simulink model "fangzhen"  (R2018b)
settings: Solver=ode45  StartTime=0.0  StopTime=10  FixedStep=0.0002  MaxStep=1/5000/25  MinStep=1/5000/100  RelTol=2e-4  EnableMultiTasking=on
libraries: powerlib_meascontrol x6, powerlib x5, simulink x4, powerlib_extras x1
(part 1 of 2)
settings Model: Creator=Administrator  LastModifiedBy=ThinkPad
settings DataIOCC: LimitDataPoints=on  SaveFormat=Array  SignalLoggingSaveFormat=ModelDataLogs
settings OptimizationCC: ExpressionDepthLimit=2147483647  LifeSpan=inf
settings DebuggingCC: UnderspecifiedInitializationDetection=Classic  MergeDetectMultiDrivingBlocksExec=none  SolverPrmCheckMsg=warning  FcnCallInpInsideContextMsg=warning  UnconnectedInputMsg=none  UnconnectedOutputMsg=none  UnconnectedLineMsg=none  StateNameClashWarn=warning  LibraryContextMissingDiagnostic=none  SFUnexpectedBacktrackingDiag=warning  SFNoUnconditionalDefaultTransitionDiag=warning  SFExecutionAtInitializationDiag=none
settings HardwareCC: ProdBitPerPointer=32  ProdBitPerSizeT=32  ProdBitPerPtrDiffT=32  ProdLargestAtomicFloat=None  ProdIntDivRoundTo=Undefined  ProdEndianess=Unspecified  ProdWordSize=32  ProdHWDeviceType=32-bit Generic
settings ModelReferenceCC: PropagateSignalLabelsOutOfModel=off
settings SFSimCC: SimUseLocalCustomCode=off
settings RTWCC: RTWUseLocalCustomCode=off
settings CodeAppCC: StateflowObjectComments=on
settings GRTTargetCC: TargetLangStandard=C89/C90 (ANSI)  GeneratePreprocessorConditionals=Disable all
settings ConfigComp: CovMetricSettings=dw  CovHtmlReporting=on  CovSaveCumulativeToWorkspaceVar=on  CovSaveSingleToWorkspaceVar=on  CovExternalEMLEnable=off
settings SimscapeCC: SimscapeNormalizeSystem=off

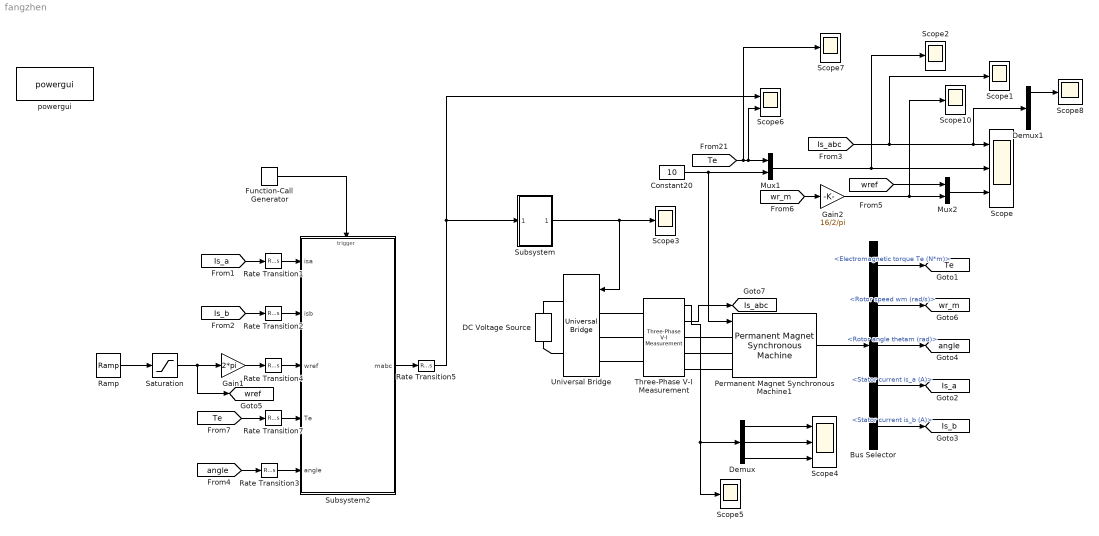
== system fangzhen ==
  Bus Selector : BusSelector  OutputSignals=Electromagnetic torque Te (N*m),Rotor speed wm (rad/s),Rotor angle thetam (rad),Stator current is_a (A),Stator current is_b (A)
  Constant20 : Constant  Value=10  OutDataTypeStr=double
  DC Voltage Source : powerlib/Electrical Sources/DC Voltage Source  Amplitude=400  Measurements=None
      settings: SourceProductName=Simscape Electrical
  Demux : Demux  Outputs=3
  Demux1 : Demux  Outputs=3
  Function-Call Generator : simulink/Ports & Subsystems/Function-Call Generator  sample_time=1/5000  numberOfIterations=1
  Gain1 : Gain  Gain=2*pi
  Gain2 : Gain  Gain=16/2/pi
  Mux1 : Mux  Inputs=2
  Mux2 : Mux  Inputs=2
  Permanent Magnet Synchronous Machine1 : powerlib/Machines/Permanent Magnet Synchronous Machine  NbPhases=3  FluxDistribution=Sinusoidal  RotorType=Round  MechanicalLoad=Torque Tm  PresetModel=No  ShowDetailedParameters=on  MeasurementBus=off  Resistance=0.4  Inductance=8.5e-3  dqInductances=[8.5e-3,8.5e-3]  La=0.004  MachineConstant=Torque Constant (N.m / A_peak)  Flux=0.56178  VoltageCst=1630.3396  TorqueCst=13.4828  Flat=120  Mechanical=[0.00062 0.0003035 16 0]  PolePairs=16  InitialConditions=[0,0, 0,0]  InitialConditions5ph=[0 0 0 0 0 0]  TsPowergui=0  TsBlock=-1  RefAngle=Aligned with phase A axis (original Park)
  Ramp : simulink/Sources/Ramp  slope=30/0.1  start=0  InitialOutput=0
  Rate Transition{1..5,7} (6 alike) : RateTransition  Integrity=off
  Saturation : Saturate  UpperLimit=10  LowerLimit=0
  Scope : Scope  NumInputPorts=3
  Scope{1..3,5,7..8,10} (7 alike) : Scope
  Scope4 : Scope  NumInputPorts=3
  Scope6 : Scope  NumInputPorts=2
  Subsystem : Subsystem
  Subsystem2 : Subsystem
  Three-Phase V-I Measurement : powerlib/Measurements/Three-Phase V-I Measurement  VoltageMeasurement=phase-to-phase  SetLabelV=off  LabelV=Vabc  Vpu=off  VpuLL=off  CurrentMeasurement=yes  SetLabelI=off  LabelI=Iabc  Ipu=off  Pbase=100e6  Vbase=500e3  OutputType=Complex  PhasorSimulation=off  PSBequivalent=0
      settings: SourceProductName=Simscape Electrical
  Universal Bridge : powerlib/Power Electronics/Universal Bridge  Arms=3  SnubberResistance=1e5  SnubberCapacitance=inf  Device=IGBT / Diodes  Ron=1e-3  Lon=0  ForwardVoltages="[  3  2  ]"  ForwardVoltage=0  GTOparameters=[ 10e-6 , 20e-6 ]  IGBTparameters=[ 1e-6 , 2e-6 ]  Measurements=All voltages and currents  Measurements_2=None  converterType=Rectifier
      settings: SourceProductName=Simscape Electrical
  powergui : powerlib/powergui  Priority=2  SimulationMode=Discrete  SampleTime=1/5000/30/20  frequency=60  Iterations=50  frequencyindice=0  Pbase=100e6  ErrMax=1e-4  UnitsV=kV  UnitsW=MW  buscounter=0  FunctionMessages=off  echomessages=off  EnableUseOfTLC=off  CurrentSourceSwitches=off  DisableSnubberDevices=off  DisableRonSwitches=off  DisableVfSwitches=off  DisplayEquations=off  SolverType=Tustin  Interpol=off  ExternalGateDelay=off  methode=off  Ts=0  x0status=blocks  SPID=off  SwTol=0  HookPort=off  RestoreLinks=warning  ResistiveCurrentMeasurement=off  Frange=[0:2:500]  Ylog=off  Xlog=on  ShowGrid=off  save=off  variable=ZData  structure=TEwu  ZoomFFT=off  StartTime=9  cycles=8  DisplayStyle=1  fundamental=10  FreqAxis=on  MaxFrequency=100  frequencyindicesteady=1  RmsSteady=1  display=off
  tag scope: Is_a=global, Is_abc=global, Is_b=global, Te=global, angle=global, wr_m=global, wref=global
  wires:
  [wref] -> Mux2/1
  Rate Transition7/1 -> Subsystem2/4(Te)
  Gain2/1 -> Mux2/2, Scope10/1
  Three-Phase V-I Measurement/2 -> [Is_abc]
  [angle] -> Rate Transition3/1
  Rate Transition2/1 -> Subsystem2/2(isb)
  Bus Selector/2 -> [wr_m]  "<Rotor speed wm (rad/s)>"
  Demux/1 -> Scope4/1
  Ramp/1 -> Saturation/1
  Demux/2 -> Scope4/2
  Gain1/1 -> Rate Transition4/1
  Bus Selector/5 -> [Is_b]  "<Stator current is_b (A)>"
  [Is_b] -> Rate Transition2/1
  Mux2/1 -> Scope/3
  Rate Transition5/1 -> Subsystem/1(In1), Scope6/1
  Rate Transition1/1 -> Subsystem2/1(isa)
  Rate Transition4/1 -> Subsystem2/3(wref)
  Bus Selector/1 -> [Te]  "<Electromagnetic torque Te (N*m)>"
  [wr_m] -> Gain2/1
  [Te] -> Scope7/1, Mux1/1, Scope6/2
  Three-Phase V-I Measurement/1 -> Demux/1, Scope5/1
  [Te] -> Rate Transition7/1
  Bus Selector/3 -> [angle]  "<Rotor angle thetam (rad)>"
  [Is_a] -> Rate Transition1/1
  Permanent Magnet Synchronous Machine1/1 -> Bus Selector/1
  Constant20/1 -> Permanent Magnet Synchronous Machine1/1, Mux1/2
  Saturation/1 -> Gain1/1, [wref]
  Mux1/1 -> Scope2/1, Scope/2
  Rate Transition3/1 -> Subsystem2/5(angle)
  Bus Selector/4 -> [Is_a]  "<Stator current is_a (A)>"
  [Is_abc] -> Scope1/1, Demux1/1, Scope/1
  Demux/3 -> Scope4/3
  Subsystem/1(Out1) -> Universal Bridge/1, Scope3/1
  Function-Call Generator/1 -> Subsystem2/Trigger
  Subsystem2/1(mabc) -> Rate Transition5/1
  Demux1/1 -> Scope8/1
  connections:
  Universal Bridge/LConn2 -- Three-Phase V-I Measurement/LConn2
  Universal Bridge/LConn3 -- Three-Phase V-I Measurement/LConn3
  Universal Bridge/LConn1 -- Three-Phase V-I Measurement/LConn1
  DC Voltage Source/RConn1 -- Universal Bridge/RConn1
  Universal Bridge/RConn2 -- DC Voltage Source/LConn1
  Permanent Magnet Synchronous Machine1/LConn2 -- Three-Phase V-I Measurement/RConn2
  Three-Phase V-I Measurement/RConn3 -- Permanent Magnet Synchronous Machine1/LConn3
  Permanent Magnet Synchronous Machine1/LConn1 -- Three-Phase V-I Measurement/RConn1

== system fangzhen/Subsystem ==
  In1 : Inport
  Demux1 : Demux  Outputs=6
  Mux : Mux  Inputs=6
  On Delay{,1..5} (6 alike) : powerlib_meascontrol/Logic/On Delay  DelayType=On delay  delay=5e-6  ic=0  Ts=0
      settings: SourceProductName=Simscape Power Systems
  PWM Generator : powerlib_extras/Control  Blocks/PWM Generator  GeneratorMode="3-arm  bridge (6 pulses)"  Fc=5000  Internal=off  mIndex=0.4  Freq=60  Phase=0
  Scope{1..3,7..9} (6 alike) : Scope  NumInputPorts=2
  Out1 : Outport
  wires:
  Demux1/6 -> On Delay5/1, Scope7/2
  Demux1/3 -> On Delay2/1, Scope8/1
  In1/1 -> PWM Generator/1
  Demux1/4 -> On Delay3/1, Scope8/2
  PWM Generator/1 -> Demux1/1
  Demux1/2 -> On Delay1/1, Scope9/2
  Demux1/5 -> On Delay4/1, Scope7/1
  Demux1/1 -> Scope9/1, On Delay/1
  On Delay/1 -> Scope3/1, Mux/1
  On Delay1/1 -> Mux/2, Scope3/2
  On Delay2/1 -> Scope2/1, Mux/3
  On Delay3/1 -> Scope2/2, Mux/4
  On Delay4/1 -> Scope1/1, Mux/5
  On Delay5/1 -> Scope1/2, Mux/6
  Mux/1 -> Out1/1

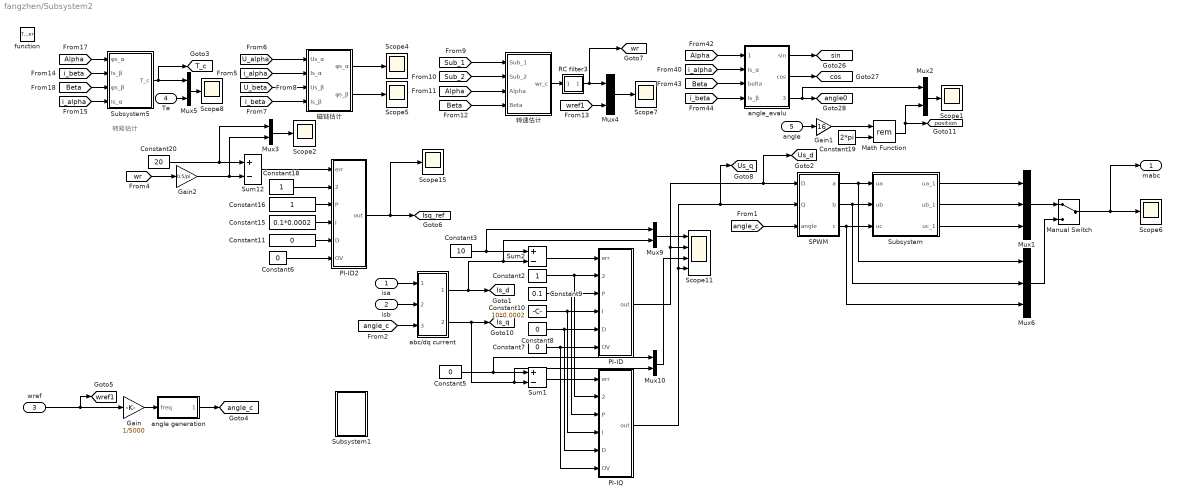
== system fangzhen/Subsystem2 ==
  note: 转矩估计
  isa : Inport
  isb : Inport  Port=2
  wref : Inport  Port=3
  Te : Inport  Port=4
  angle : Inport  Port=5
  function : TriggerPort  TriggerType=function-call  VariantControl=(inherit)
  Constant10 : Constant  Value=10*0.0002  OutDataTypeStr=double
  Constant{5..8,11} (5 alike) : Constant  Value=0  OutDataTypeStr=double
  Constant15 : Constant  Value=0.1*0.0002  OutDataTypeStr=double
  Constant16 : Constant  OutDataTypeStr=double
  Constant18 : Constant  OutDataTypeStr=double
  Constant19 : Constant  Value=2*pi  OutDataTypeStr=double
  Constant2 : Constant  OutDataTypeStr=double
  Constant20 : Constant  Value=20  OutDataTypeStr=double
  Constant3 : Constant  Value=10  OutDataTypeStr=double
  Constant9 : Constant  Value=0.1  OutDataTypeStr=double
  Gain : Gain  Gain=1/5000
  Gain1 : Gain  Gain=16
  Gain2 : Gain  Gain=0.5/pi
  Manual Switch : ManualSwitch
  Math Function : Math  Operator=rem  SaturateOnIntegerOverflow=on
  Mux1 : Mux  Inputs=3
  Mux{2..5,9..10} (6 alike) : Mux  Inputs=2
  Mux6 : Mux  Inputs=3
  PI-ID : Subsystem  mask{ermax=1000, ermin=-1000, max=1, min=-1}
      mask prompts: ermax "Err max limit"; ermin "Err min limit"; max "Output max limit"; min "Output min limit"
  PI-ID2 : Subsystem  mask{ermax=10, ermin=-10, max=5, min=0}
      mask prompts: ermax "Err max limit"; ermin "Err min limit"; max "Output max limit"; min "Output min limit"
  PI-IQ : Subsystem  mask{ermax=100, ermin=-100, max=1, min=-1}
      mask prompts: ermax "Err max limit"; ermin "Err min limit"; max "Output max limit"; min "Output min limit"
  RC filter3 : Subsystem  mask{a=1/4}
      mask prompts: a "Time Constant"
  SPWM : Subsystem
  Scope{1..2,4..8,15} (8 alike) : Scope
  Scope11 : Scope  NumInputPorts=4
  Subsystem : Subsystem
  Subsystem1 : Subsystem
  Subsystem5 : Subsystem
  Sum1 : Sum  Inputs=+-
  Sum12 : Sum  Inputs=+-
  Sum2 : Sum  Inputs=+-
  abc/dq current : Subsystem
  angle generation : Subsystem
  angle_evalu : Subsystem
  磁链估计 : Subsystem
  转速估计 : Subsystem
  mabc : Outport
  tag scope: Is_d=global, Is_q=global, Isq_ref=global, T_c=global, Us_d=global, Us_q=global, angle0=global, angle_c=global, cos=global, position=global, sin=global, wr=global, wref1=global
  wires:
  Mux1/1 -> Manual Switch/1
  isa/1 -> abc/dq current/1(iga)
  abc/dq current/1(igd) -> Sum2/2, Mux9/2, [Is_d]
  abc/dq current/2(igq) -> Sum1/2, Mux10/2, [Is_q]
  Constant7/1 -> PI-ID/6(OV), PI-IQ/6(OV)
  Constant8/1 -> PI-ID/5(D), PI-IQ/5(D)
  Constant10/1 -> PI-ID/4(I), PI-IQ/4(I)
  Constant9/1 -> PI-ID/3(P), PI-IQ/3(P)
  Sum2/1 -> PI-ID/1(err)
  Constant2/1 -> PI-ID/2(reset), PI-IQ/2(reset)
  PI-ID/1(out) -> Scope11/2, [Us_d], SPWM/1(D)
  PI-IQ/1(out) -> Scope11/4, [Us_q], SPWM/2(Q)
  Sum1/1 -> PI-IQ/1(err)
  [angle_c] -> SPWM/3(angle)
  Gain/1 -> angle generation/1(freq)
  Mux9/1 -> Scope11/1
  Mux10/1 -> Scope11/3
  isb/1 -> abc/dq current/2(igb)
  angle generation/1(angle_0) -> [angle_c]
  [angle_c] -> abc/dq current/3(angle)
  wref/1 -> Gain/1, [wref1]
  [Beta] -> 转速估计/4(Beta)
  [Alpha] -> 转速估计/3(Alpha)
  [Sub_2] -> 转速估计/2(Sub_2)
  [Sub_1] -> 转速估计/1(Sub_1)
  转速估计/1(wr_c) -> RC filter3/1(x)
  Mux4/1 -> Scope7/1
  [U_alpha] -> 磁链估计/1(Us_α)
  [i_alpha] -> 磁链估计/2(Is_α)
  [U_beta] -> 磁链估计/3(Us_β)
  [i_beta] -> 磁链估计/4(Is_β)
  磁链估计/2(φs_β) -> Scope5/1
  磁链估计/1(φs_α) -> Scope4/1
  [Alpha] -> Subsystem5/1(φs_α)
  [Beta] -> Subsystem5/3(φs_β)
  [i_beta] -> Subsystem5/2(Is_β)
  [i_alpha] -> Subsystem5/4(Is_α)
  Subsystem5/1(T_c) -> Mux5/1, [T_c]
  Mux5/1 -> Scope8/1
  Te/1 -> Mux5/2
  RC filter3/1(y) -> [wr], Mux4/1
  [wref1] -> Mux4/2
  [wr] -> Gain2/1
  Constant20/1 -> Sum12/1, Mux3/1
  Sum12/1 -> PI-ID2/1(err)
  Constant18/1 -> PI-ID2/2(reset)
  Constant16/1 -> PI-ID2/3(P)
  Constant15/1 -> PI-ID2/4(I)
  Constant11/1 -> PI-ID2/5(D)
  Constant6/1 -> PI-ID2/6(OV)
  PI-ID2/1(out) -> Scope15/1, [Isq_ref]
  Constant5/1 -> Sum1/1, Mux10/1
  Constant3/1 -> Sum2/1, Mux9/1
  [Alpha] -> angle_evalu/1(alpha)
  [Beta] -> angle_evalu/3(belta)
  [i_beta] -> angle_evalu/4(Is_β)
  [i_alpha] -> angle_evalu/2(Is_α)
  angle_evalu/1(sin) -> [sin]
  angle_evalu/2(cos) -> [cos]
  angle_evalu/3(angle_0) -> [angle0], Mux2/1
  Mux2/1 -> Scope1/1
  angle/1 -> Gain1/1
  Mux3/1 -> Scope2/1
  Constant19/1 -> Math Function/2
  Gain1/1 -> Math Function/1
  Math Function/1 -> Mux2/2, [position]
  Gain2/1 -> Sum12/2, Mux3/2
  SPWM/1(a) -> Subsystem/1(ua), Mux6/1
  SPWM/2(b) -> Subsystem/2(ub), Mux6/2
  SPWM/3(c) -> Subsystem/3(uc), Mux6/3
  Subsystem/1(ua_1) -> Mux1/1
  Subsystem/3(uc_1) -> Mux1/3
  Subsystem/2(ub_1) -> Mux1/2
  Mux6/1 -> Manual Switch/2
  Manual Switch/1 -> Scope6/1, mabc/1

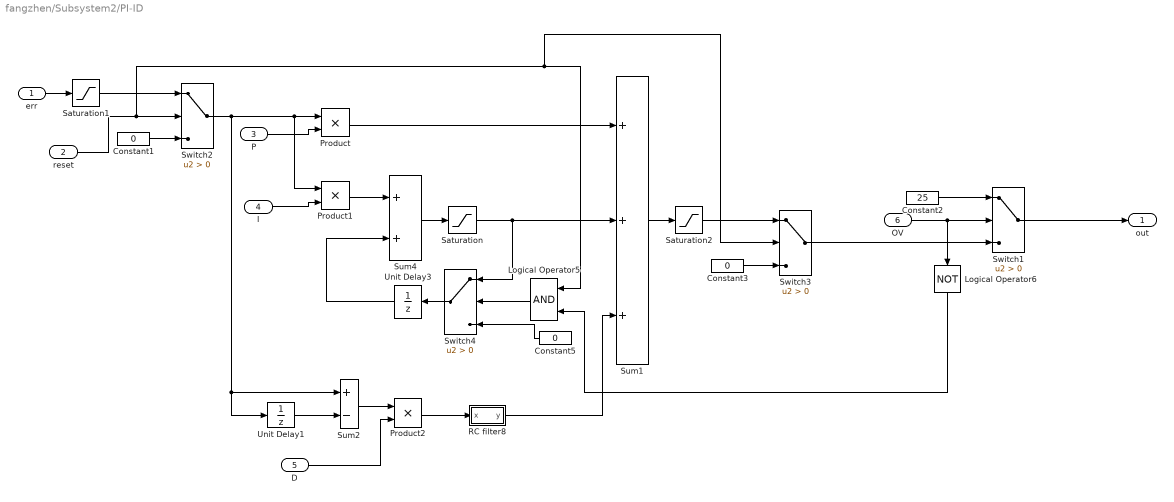
== system fangzhen/Subsystem2/PI-ID ==
  err : Inport
  reset : Inport  Port=2
  P : Inport  Port=3
  I : Inport  Port=4
  D : Inport  Port=5
  OV : Inport  Port=6
  Constant1 : Constant  Value=0  OutDataTypeStr=Inherit: Inherit via back propagation
  Constant2 : Constant  Value=25  OutDataTypeStr=Inherit: Inherit via back propagation
  Constant3 : Constant  Value=0  OutDataTypeStr=Inherit: Inherit via back propagation
  Constant5 : Constant  Value=0  OutDataTypeStr=Inherit: Inherit via back propagation
  Logical Operator5 : Logic  AllPortsSameDT=off  OutDataTypeStr=boolean
  Logical Operator6 : Logic  Operator=NOT  AllPortsSameDT=off  OutDataTypeStr=boolean
  Product : Product  RndMeth=Zero
  Product1 : Product  RndMeth=Zero
  Product2 : Product  RndMeth=Zero
  RC filter8 : Subsystem  mask{a=0.4}
      mask prompts: a "Time Constant"
  Saturation : Saturate  UpperLimit=max  LowerLimit=min  LinearizeAsGain=off  ZeroCross=off  OutDataTypeStr=double
  Saturation1 : Saturate  UpperLimit=ermax  LowerLimit=ermin  LinearizeAsGain=off  ZeroCross=off  OutDataTypeStr=double
  Saturation2 : Saturate  UpperLimit=max  LowerLimit=min  LinearizeAsGain=off  ZeroCross=off  OutDataTypeStr=double
  Sum1 : Sum  Inputs=+++
  Sum2 : Sum  Inputs=+-
  Sum4 : Sum
  Switch{1..4} (4 alike) : Switch  Criteria=u2 > Threshold  SaturateOnIntegerOverflow=on  InputSameDT=on
  Unit Delay1 : UnitDelay  SampleTime=-1
  Unit Delay3 : UnitDelay  SampleTime=-1
  out : Outport
  wires:
  Logical Operator6/1 -> Logical Operator5/2
  Logical Operator5/1 -> Switch4/2
  RC filter8/1(y) -> Sum1/3
  Constant3/1 -> Switch3/3
  Switch3/1 -> Switch1/3
  Saturation2/1 -> Switch3/1
  Switch1/1 -> out/1
  OV/1 -> Logical Operator6/1, Switch1/2
  Constant2/1 -> Switch1/1
  Sum1/1 -> Saturation2/1
  Product2/1 -> RC filter8/1(x)
  Unit Delay1/1 -> Sum2/2
  D/1 -> Product2/2
  Sum2/1 -> Product2/1
  Switch4/1 -> Unit Delay3/1
  Unit Delay3/1 -> Sum4/2
  Saturation/1 -> Switch4/1, Sum1/2
  Sum4/1 -> Saturation/1
  Product1/1 -> Sum4/1
  I/1 -> Product1/2
  Product/1 -> Sum1/1
  Saturation1/1 -> Switch2/1
  err/1 -> Saturation1/1
  Constant1/1 -> Switch2/3
  reset/1 -> Logical Operator5/1, Switch3/2, Switch2/2
  Switch2/1 -> Unit Delay1/1, Sum2/1, Product1/1, Product/1
  P/1 -> Product/2
  Constant5/1 -> Switch4/3

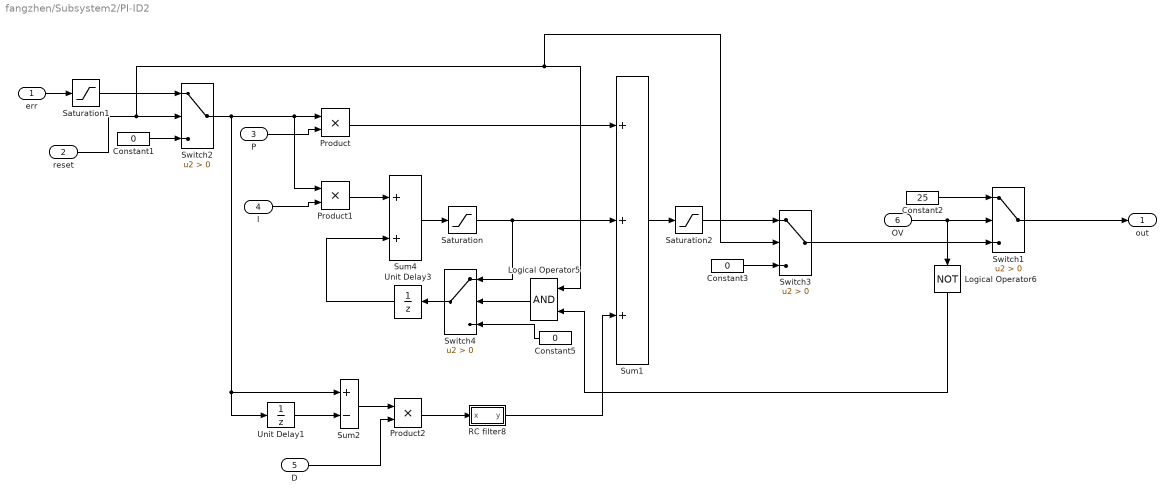
== system fangzhen/Subsystem2/PI-ID2 ==
  err : Inport
  reset : Inport  Port=2
  P : Inport  Port=3
  I : Inport  Port=4
  D : Inport  Port=5
  OV : Inport  Port=6
  Constant1 : Constant  Value=0  OutDataTypeStr=Inherit: Inherit via back propagation
  Constant2 : Constant  Value=25  OutDataTypeStr=Inherit: Inherit via back propagation
  Constant3 : Constant  Value=0  OutDataTypeStr=Inherit: Inherit via back propagation
  Constant5 : Constant  Value=0  OutDataTypeStr=Inherit: Inherit via back propagation
  Logical Operator5 : Logic  AllPortsSameDT=off  OutDataTypeStr=boolean
  Logical Operator6 : Logic  Operator=NOT  AllPortsSameDT=off  OutDataTypeStr=boolean
  Product : Product  RndMeth=Zero
  Product1 : Product  RndMeth=Zero
  Product2 : Product  RndMeth=Zero
  RC filter8 : Subsystem  mask{a=0.4}
      mask prompts: a "Time Constant"
  Saturation : Saturate  UpperLimit=max  LowerLimit=min  LinearizeAsGain=off  ZeroCross=off  OutDataTypeStr=double
  Saturation1 : Saturate  UpperLimit=ermax  LowerLimit=ermin  LinearizeAsGain=off  ZeroCross=off  OutDataTypeStr=double
  Saturation2 : Saturate  UpperLimit=max  LowerLimit=min  LinearizeAsGain=off  ZeroCross=off  OutDataTypeStr=double
  Sum1 : Sum  Inputs=+++
  Sum2 : Sum  Inputs=+-
  Sum4 : Sum
  Switch{1..4} (4 alike) : Switch  Criteria=u2 > Threshold  SaturateOnIntegerOverflow=on  InputSameDT=on
  Unit Delay1 : UnitDelay  SampleTime=-1
  Unit Delay3 : UnitDelay  SampleTime=-1
  out : Outport
  wires:
  Constant5/1 -> Switch4/3
  P/1 -> Product/2
  Switch2/1 -> Product/1, Product1/1, Sum2/1, Unit Delay1/1
  reset/1 -> Switch2/2, Switch3/2, Logical Operator5/1
  Constant1/1 -> Switch2/3
  err/1 -> Saturation1/1
  Saturation1/1 -> Switch2/1
  Product/1 -> Sum1/1
  I/1 -> Product1/2
  Product1/1 -> Sum4/1
  Sum4/1 -> Saturation/1
  Saturation/1 -> Sum1/2, Switch4/1
  Unit Delay3/1 -> Sum4/2
  Switch4/1 -> Unit Delay3/1
  Sum2/1 -> Product2/1
  D/1 -> Product2/2
  Unit Delay1/1 -> Sum2/2
  Product2/1 -> RC filter8/1(x)
  Sum1/1 -> Saturation2/1
  Constant2/1 -> Switch1/1
  OV/1 -> Switch1/2, Logical Operator6/1
  Switch1/1 -> out/1
  Saturation2/1 -> Switch3/1
  Switch3/1 -> Switch1/3
  Constant3/1 -> Switch3/3
  RC filter8/1(y) -> Sum1/3
  Logical Operator5/1 -> Switch4/2
  Logical Operator6/1 -> Logical Operator5/2

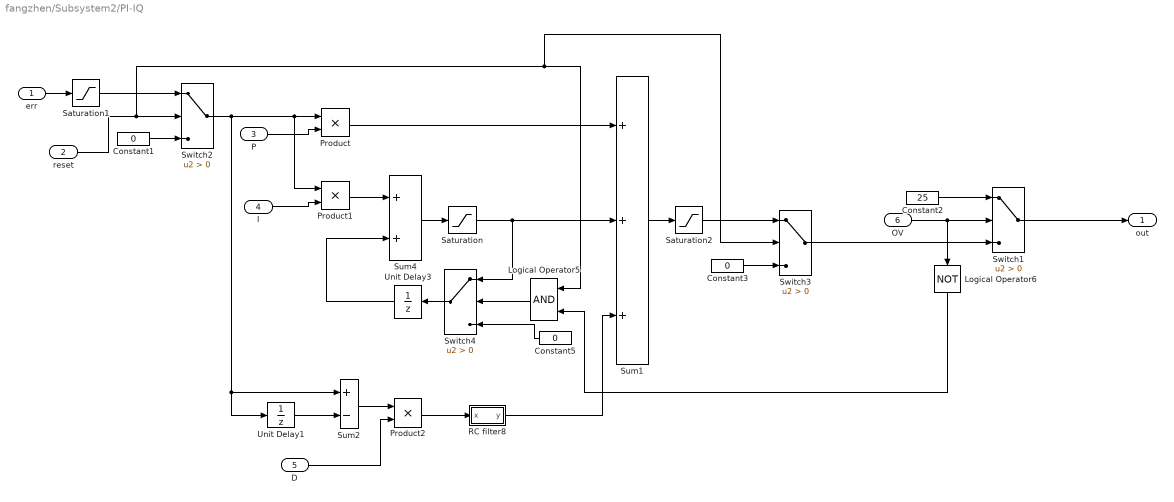
== system fangzhen/Subsystem2/PI-IQ ==
  err : Inport
  reset : Inport  Port=2
  P : Inport  Port=3
  I : Inport  Port=4
  D : Inport  Port=5
  OV : Inport  Port=6
  Constant1 : Constant  Value=0  OutDataTypeStr=Inherit: Inherit via back propagation
  Constant2 : Constant  Value=25  OutDataTypeStr=Inherit: Inherit via back propagation
  Constant3 : Constant  Value=0  OutDataTypeStr=Inherit: Inherit via back propagation
  Constant5 : Constant  Value=0  OutDataTypeStr=Inherit: Inherit via back propagation
  Logical Operator5 : Logic  AllPortsSameDT=off  OutDataTypeStr=boolean
  Logical Operator6 : Logic  Operator=NOT  AllPortsSameDT=off  OutDataTypeStr=boolean
  Product : Product  RndMeth=Zero
  Product1 : Product  RndMeth=Zero
  Product2 : Product  RndMeth=Zero
  RC filter8 : Subsystem  mask{a=0.4}
      mask prompts: a "Time Constant"
  Saturation : Saturate  UpperLimit=max  LowerLimit=min  LinearizeAsGain=off  ZeroCross=off  OutDataTypeStr=double
  Saturation1 : Saturate  UpperLimit=ermax  LowerLimit=ermin  LinearizeAsGain=off  ZeroCross=off  OutDataTypeStr=double
  Saturation2 : Saturate  UpperLimit=max  LowerLimit=min  LinearizeAsGain=off  ZeroCross=off  OutDataTypeStr=double
  Sum1 : Sum  Inputs=+++
  Sum2 : Sum  Inputs=+-
  Sum4 : Sum
  Switch{1..4} (4 alike) : Switch  Criteria=u2 > Threshold  SaturateOnIntegerOverflow=on  InputSameDT=on
  Unit Delay1 : UnitDelay  SampleTime=-1
  Unit Delay3 : UnitDelay  SampleTime=-1
  out : Outport
  wires:
  Constant5/1 -> Switch4/3
  P/1 -> Product/2
  Switch2/1 -> Product/1, Product1/1, Sum2/1, Unit Delay1/1
  reset/1 -> Switch2/2, Switch3/2, Logical Operator5/1
  Constant1/1 -> Switch2/3
  err/1 -> Saturation1/1
  Saturation1/1 -> Switch2/1
  Product/1 -> Sum1/1
  I/1 -> Product1/2
  Product1/1 -> Sum4/1
  Sum4/1 -> Saturation/1
  Saturation/1 -> Sum1/2, Switch4/1
  Unit Delay3/1 -> Sum4/2
  Switch4/1 -> Unit Delay3/1
  Sum2/1 -> Product2/1
  D/1 -> Product2/2
  Unit Delay1/1 -> Sum2/2
  Product2/1 -> RC filter8/1(x)
  Sum1/1 -> Saturation2/1
  Constant2/1 -> Switch1/1
  OV/1 -> Switch1/2, Logical Operator6/1
  Switch1/1 -> out/1
  Saturation2/1 -> Switch3/1
  Switch3/1 -> Switch1/3
  Constant3/1 -> Switch3/3
  RC filter8/1(y) -> Sum1/3
  Logical Operator5/1 -> Switch4/2
  Logical Operator6/1 -> Logical Operator5/2

== system fangzhen/Subsystem2/RC filter3 ==
  x : Inport
  Constant2 : Constant  Value=a  OutDataTypeStr=double
  Constant3 : Constant  Value=1-a  OutDataTypeStr=double
  Divide : Product
  Divide1 : Product
  Sum2 : Sum
  Unit Delay2 : UnitDelay  SampleTime=-1
  y : Outport
  wires:
  Unit Delay2/1 -> Divide1/2
  Sum2/1 -> Unit Delay2/1, y/1
  Divide1/1 -> Sum2/2
  Divide/1 -> Sum2/1
  Constant3/1 -> Divide1/1
  Constant2/1 -> Divide/2
  x/1 -> Divide/1

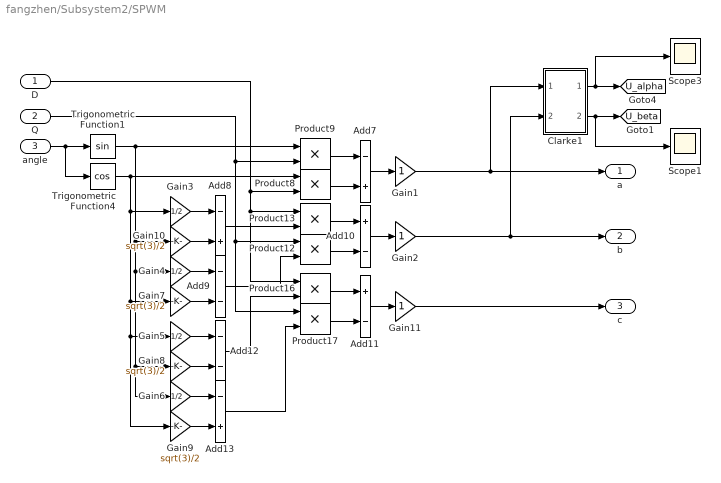
== system fangzhen/Subsystem2/SPWM ==
  D : Inport
  Q : Inport  Port=2
  angle : Inport  Port=3
  Add10 : Sum  Inputs=+-
  Add11 : Sum  Inputs=+-
  Add12 : Sum  Inputs=--
  Add13 : Sum  Inputs=-+
  Add7 : Sum  Inputs=-+
  Add8 : Sum  Inputs=-+
  Add9 : Sum  Inputs=--
  Clarke1 : Subsystem
  Gain1 : Gain
  Gain{7..10} (4 alike) : Gain  Gain=sqrt(3)/2
  Gain11 : Gain
  Gain2 : Gain
  Gain{3..6} (4 alike) : Gain  Gain=1/2
  Product{8..9,12..13,16..17} (6 alike) : Product  RndMeth=Zero
  Scope1 : Scope
  Scope3 : Scope
  Trigonometric Function1 : Trigonometry
  Trigonometric Function4 : Trigonometry  Operator=cos
  a : Outport
  b : Outport  Port=2
  c : Outport  Port=3
  tag scope: U_alpha=global, U_beta=global
  wires:
  angle/1 -> Trigonometric Function1/1, Trigonometric Function4/1
  Trigonometric Function4/1 -> Product8/1, Gain3/1, Gain5/1, Gain9/1, Gain7/1
  Product8/1 -> Add7/2
  Trigonometric Function1/1 -> Product9/1, Gain4/1, Gain6/1, Gain8/1, Gain10/1
  Product9/1 -> Add7/1
  Gain3/1 -> Add8/1
  Gain4/1 -> Add9/1
  Gain7/1 -> Add9/2
  Product13/1 -> Add10/1
  Product12/1 -> Add10/2
  Add8/1 -> Product13/2
  Add9/1 -> Product12/2
  Product16/1 -> Add11/1
  Product17/1 -> Add11/2
  Add12/1 -> Product16/2
  Add13/1 -> Product17/2
  Add7/1 -> Gain1/1
  Add10/1 -> Gain2/1
  Add11/1 -> Gain11/1
  Gain6/1 -> Add13/1
  Gain8/1 -> Add12/2
  Gain5/1 -> Add12/1
  Gain9/1 -> Add13/2
  Gain10/1 -> Add8/2
  D/1 -> Product8/2, Product13/1, Product16/1
  Q/1 -> Product9/2, Product12/1, Product17/1
  Gain1/1 -> a/1, Clarke1/1(In1)
  Gain2/1 -> b/1, Clarke1/2(In2)
  Gain11/1 -> c/1
  Clarke1/1(alpha) -> [U_alpha], Scope3/1
  Clarke1/2(beta) -> [U_beta], Scope1/1

== system fangzhen/Subsystem2/Subsystem ==
  ua : Inport
  ub : Inport  Port=2
  uc : Inport  Port=3
  Scope6 : Scope  NumInputPorts=2
  Sum4 : Sum  Inputs=+++
  Sum5 : Sum  Inputs=+++
  Sum6 : Sum  Inputs=+++
  ua_1 : Outport
  ub_1 : Outport  Port=2
  uc_1 : Outport  Port=3
  wires:
  [uc_7] -> Sum6/2
  [uc_5] -> Sum6/1
  [ub_7] -> Sum5/2
  ub/1 -> Sum5/3
  uc/1 -> Sum6/3
  [ub_5] -> Sum5/1
  [ua_7] -> Scope6/2, Sum4/2
  [ua_5] -> Sum4/1, Scope6/1
  ua/1 -> Sum4/3
  Sum4/1 -> ua_1/1
  Sum5/1 -> ub_1/1
  Sum6/1 -> uc_1/1

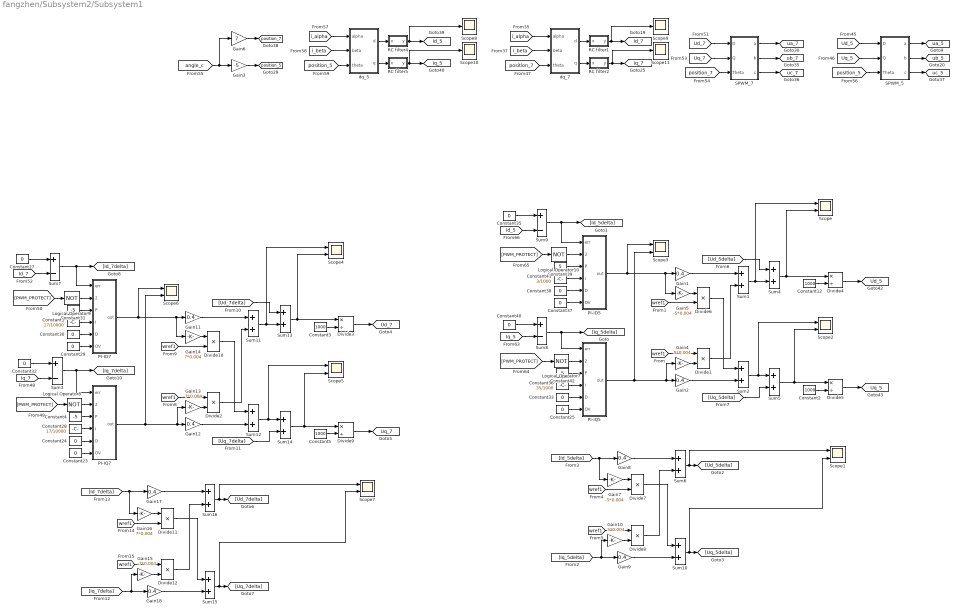
== system fangzhen/Subsystem2/Subsystem1 ==
  Constant1 : Constant  Value=17/10000  OutDataTypeStr=double
  Constant{2..3,5,12} (4 alike) : Constant  Value=1000  OutDataTypeStr=double
  Constant{23..25,27,29..30,32..33,35,37..38,40} (12 alike) : Constant  Value=0  OutDataTypeStr=double
  Constant28 : Constant  Value=17/10000  OutDataTypeStr=double
  Constant31 : Constant  Value=-5  OutDataTypeStr=double
  Constant36 : Constant  Value=35/1000  OutDataTypeStr=double
  Constant39 : Constant  Value=5  OutDataTypeStr=double
  Constant4 : Constant  Value=-5  OutDataTypeStr=double
  Constant41 : Constant  Value=3/1000  VectorParams1D=off  OutDataTypeStr=double
  Constant42 : Constant  Value=5  OutDataTypeStr=double
  Divide{1..2,6..8,10..12} (8 alike) : Product  Inputs=**
  Divide{3..5,9} (4 alike) : Product  Inputs=*/
  Gain{1..2,8..9,11..12,17..18} (8 alike) : Gain  Gain=0.4
  Gain10 : Gain  Gain=5*0.004
  Gain13 : Gain  Gain=-7*0.004
  Gain14 : Gain  Gain=7*0.004
  Gain15 : Gain  Gain=-7*0.004
  Gain16 : Gain  Gain=7*0.004
  Gain3 : Gain  Gain=-5
  Gain4 : Gain  Gain=5*0.004
  Gain5 : Gain  Gain=-5*0.004
  Gain6 : Gain  Gain=7
  Gain7 : Gain  Gain=-5*0.004
  Logical Operator{7..10} (4 alike) : Logic  Operator=NOT  AllPortsSameDT=off  OutDataTypeStr=boolean
  PI-ID5 : Subsystem  mask{ermax=3, ermin=-3, max=500, min=-500}
      mask prompts: ermax "Err max limit"; ermin "Err min limit"; max "Output max limit"; min "Output min limit"
  PI-ID7 : Subsystem  mask{ermax=3, ermin=-3, max=500, min=-500}
      mask prompts: ermax "Err max limit"; ermin "Err min limit"; max "Output max limit"; min "Output min limit"
  PI-IQ5 : Subsystem  mask{ermax=3, ermin=-3, max=500, min=-500}
      mask prompts: ermax "Err max limit"; ermin "Err min limit"; max "Output max limit"; min "Output min limit"
  PI-IQ7 : Subsystem  mask{ermax=3, ermin=-3, max=500, min=-500}
      mask prompts: ermax "Err max limit"; ermin "Err min limit"; max "Output max limit"; min "Output min limit"
  RC filter1 : Subsystem  mask{a=0.005}
      mask prompts: a "Time Constant"
  RC filter2 : Subsystem  mask{a=0.005}
      mask prompts: a "Time Constant"
  RC filter4 : Subsystem  mask{a=0.005}
      mask prompts: a "Time Constant"
  RC filter5 : Subsystem  mask{a=0.005}
      mask prompts: a "Time Constant"
  SPWM_5 : Subsystem
  SPWM_7 : Subsystem
  Scope{,1..7} (8 alike) : Scope  NumInputPorts=2
  Scope{8..11} (4 alike) : Scope
  Sum{1..2,4..6,10..16} (12 alike) : Sum
  Sum{3,7..9} (4 alike) : Sum  Inputs=+-
  dq_5 : Subsystem
  dq_7 : Subsystem
  tag scope: Id_5=global, Id_7=global, Iq_5=global, Iq_7=global, Ud_5=global, Ud_7=global, Uq_5=global, Uq_7=global, position_5=global, position_7=global, ua_5=global, ua_7=global, ub_5=global, ub_7=global, uc_5=global, uc_7=global
  wires:
  Constant29/1 -> PI-ID7/6(OV)
  [i_alpha] -> dq_7/1(alpha)
  [angle_c] -> Gain3/1, Gain6/1
  Constant27/1 -> Sum7/1
  SPWM_7/3(c) -> [uc_7]
  Gain6/1 -> [position_7]
  SPWM_5/2(b) -> [ub_5]
  [Id_7] -> Sum7/2
  Constant35/1 -> Sum9/1
  [Iq_7] -> Sum3/2
  dq_5/2(q) -> RC filter5/1(x)
  [position_7] -> SPWM_7/3(Theta)
  Constant31/1 -> PI-ID7/3(P)
  dq_7/2(q) -> RC filter2/1(x)
  Constant23/1 -> PI-IQ7/6(OV)
  RC filter2/1(y) -> Scope11/1, [Iq_7]
  [i_alpha] -> dq_5/1(alpha)
  Constant24/1 -> PI-IQ7/5(D)
  Logical Operator7/1 -> PI-IQ5/2(reset)
  SPWM_7/1(a) -> [ua_7]
  Constant25/1 -> PI-IQ5/6(OV)
  Gain3/1 -> [position_5]
  RC filter5/1(y) -> Scope10/1, [Iq_5]
  Constant40/1 -> Sum8/1
  Constant30/1 -> PI-ID7/5(D)
  RC filter1/1(y) -> Scope9/1, [Id_7]
  Sum7/1 -> PI-ID7/1(err), [Id_7delta]
  Sum9/1 -> [Id_5delta], PI-ID5/1(err)
  Constant33/1 -> PI-IQ5/5(D)
  [Ud_5] -> SPWM_5/1(D)
  [Id_5] -> Sum9/2
  Constant38/1 -> PI-ID5/5(D)
  Constant1/1 -> PI-ID7/4(I)
  PI-ID5/1(out) -> Scope3/1, Gain5/1, Gain1/1
  Logical Operator8/1 -> PI-IQ7/2(reset)
  Constant36/1 -> PI-IQ5/4(I)
  [Ud_7] -> SPWM_7/1(D)
  [PWM_PROTECT] -> Logical Operator8/1
  Sum3/1 -> [Iq_7delta], PI-IQ7/1(err)
  SPWM_7/2(b) -> [ub_7]
  dq_7/1(d) -> RC filter1/1(x)
  [position_5] -> SPWM_5/3(Theta)
  SPWM_5/1(a) -> [ua_5]
  [position_5] -> dq_5/3(theta)
  [Iq_5] -> Sum8/2
  SPWM_5/3(c) -> [uc_5]
  PI-IQ5/1(out) -> Scope3/2, Gain4/1, Gain2/1
  Constant37/1 -> PI-ID5/6(OV)
  [Uq_5] -> SPWM_5/2(Q)
  [Uq_7] -> SPWM_7/2(Q)
  [i_beta] -> dq_7/2(beta)
  Constant32/1 -> Sum3/1
  RC filter4/1(y) -> Scope8/1, [Id_5]
  [PWM_PROTECT] -> Logical Operator9/1
  [PWM_PROTECT] -> Logical Operator10/1
  [position_7] -> dq_7/3(theta)
  [i_beta] -> dq_5/2(beta)
  dq_5/1(d) -> RC filter4/1(x)
  Logical Operator9/1 -> PI-ID7/2(reset)
  [PWM_PROTECT] -> Logical Operator7/1
  Sum8/1 -> [Iq_5delta], PI-IQ5/1(err)
  Logical Operator10/1 -> PI-ID5/2(reset)
  Constant28/1 -> PI-IQ7/4(I)
  Constant41/1 -> PI-ID5/4(I)
  Constant39/1 -> PI-ID5/3(P)
  Constant4/1 -> PI-IQ7/3(P)
  Constant42/1 -> PI-IQ5/3(P)
  Gain4/1 -> Divide1/2
  [wref1] -> Divide1/1
  Gain5/1 -> Divide6/1
  [wref1] -> Divide6/2
  Gain1/1 -> Sum1/1
  Gain2/1 -> Sum2/2
  Divide6/1 -> Sum2/1
  Divide1/1 -> Sum1/2
  Sum1/1 -> Scope/1, Sum4/2
  Sum2/1 -> Scope2/1, Sum5/1
  [Id_5delta] -> Gain8/1, Gain7/1
  [wref1] -> Divide7/2
  Gain7/1 -> Divide7/1
  [wref1] -> Divide8/1
  Gain10/1 -> Divide8/2
  [Iq_5delta] -> Gain9/1, Gain10/1
  Gain8/1 -> Sum6/1
  Divide8/1 -> Sum6/2
  Gain9/1 -> Sum10/2
  Divide7/1 -> Sum10/1
  Sum6/1 -> Scope1/1, [Ud_5delta]
  Sum10/1 -> Scope1/2, [Uq_5delta]
  [Ud_5delta] -> Sum4/1
  [Uq_5delta] -> Sum5/2
  Sum4/1 -> Divide4/1, Scope/2
  Constant12/1 -> Divide4/2
  Divide4/1 -> [Ud_5]
  Sum5/1 -> Scope2/2, Divide5/1
  Constant2/1 -> Divide5/2
  Divide5/1 -> [Uq_5]
  [Uq_7delta] -> Sum14/2
  Sum11/1 -> Scope4/1, Sum13/2
  Gain14/1 -> Divide10/1
  Constant3/1 -> Divide3/2
  Sum14/1 -> Scope5/2, Divide9/1
  Sum12/1 -> Scope5/1, Sum14/1
  Constant5/1 -> Divide9/2
  [wref1] -> Divide10/2
  Divide9/1 -> [Uq_7]
  [wref1] -> Divide2/1
  [Ud_7delta] -> Sum13/1
  Divide3/1 -> [Ud_7]
  PI-IQ7/1(out) -> Scope6/2, Gain13/1, Gain12/1
  Gain13/1 -> Divide2/2
  PI-ID7/1(out) -> Scope6/1, Gain14/1, Gain11/1
  Gain11/1 -> Sum11/1
  Gain12/1 -> Sum12/2
  Divide2/1 -> Sum11/2
  Divide10/1 -> Sum12/1
  Sum13/1 -> Divide3/1, Scope4/2
  Sum15/1 -> Scope7/2, [Uq_7delta]
  Sum16/1 -> [Ud_7delta], Scope7/1
  Divide11/1 -> Sum15/1
  Gain18/1 -> Sum15/2
  Divide12/1 -> Sum16/2
  Gain17/1 -> Sum16/1
  [Iq_7delta] -> Gain15/1, Gain18/1
  Gain15/1 -> Divide12/2
  [wref1] -> Divide12/1
  Gain16/1 -> Divide11/1
  [wref1] -> Divide11/2
  [Id_7delta] -> Gain16/1, Gain17/1

== system fangzhen/Subsystem2/Subsystem5 ==
  φs_α : Inport
  Is_β : Inport  Port=2
  φs_β : Inport  Port=3
  Is_α : Inport  Port=4
  3/2*np : Gain  Gain=3/2*16
  Add : Sum  Inputs=+-
  Product1 : Product  RndMeth=Zero
  Product2 : Product  RndMeth=Zero
  Scope : Scope
  Scope1 : Scope
  Scope2 : Scope
  T_c : Outport
  wires:
  3/2*np/1 -> T_c/1
  Is_β/1 -> Product1/2
  φs_α/1 -> Product1/1
  Is_α/1 -> Product2/2
  φs_β/1 -> Product2/1
  Product1/1 -> Add/1, Scope1/1
  Product2/1 -> Add/2, Scope2/1
  Add/1 -> 3/2*np/1, Scope/1

== system fangzhen/Subsystem2/abc//dq current ==
  iga : Inport
  igb : Inport  Port=2
  angle : Inport  Port=3
  Clarke1 : Subsystem
  Park1 : Subsystem
  Scope1 : Scope
  Scope3 : Scope
  igd : Outport
  igq : Outport  Port=2
  tag scope: i_alpha=global, i_beta=global
  wires:
  Park1/1(d) -> igd/1
  iga/1 -> Clarke1/1(In1)
  Park1/2(q) -> igq/1
  igb/1 -> Clarke1/2(In2)
  Clarke1/1(alpha) -> Park1/1(alpha), [i_alpha], Scope1/1
  Clarke1/2(beta) -> Park1/2(beta), Scope3/1, [i_beta]
  angle/1 -> Park1/3(theta)

== system fangzhen/Subsystem2/angle generation ==
  freq : Inport
  Com : simulink/Logic and Bit Operations/Compare To Constant  relop=>=  const=2*pi  OutDataTypeStr=boolean
  Constant3 : Constant  Value=2*pi  OutDataTypeStr=double
  Rem : Math  Operator=rem  SaturateOnIntegerOverflow=on
  Sum11 : Sum
  Switch2 : Switch  Threshold=1
  Unit Delay1 : UnitDelay  SampleTime=-1
  angle_0 : Outport
  wires:
  Unit Delay1/1 -> Sum11/1
  freq/1 -> Sum11/2
  Sum11/1 -> Com/1, Switch2/3, Rem/1
  Switch2/1 -> angle_0/1, Unit Delay1/1
  Com/1 -> Switch2/2
  Rem/1 -> Switch2/1
  Constant3/1 -> Rem/2

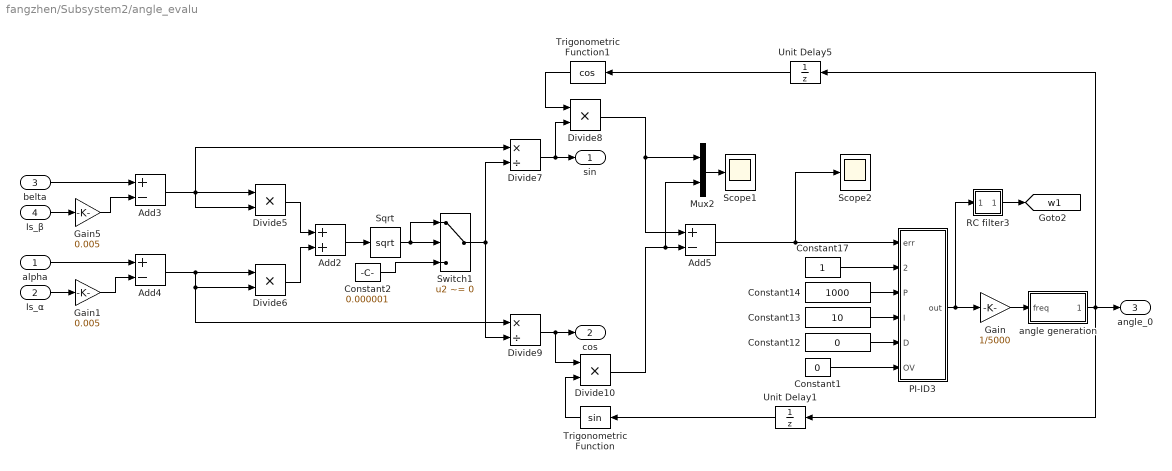
== system fangzhen/Subsystem2/angle_evalu ==
  alpha : Inport
  Is_α : Inport  Port=2
  belta : Inport  Port=3
  Is_β : Inport  Port=4
  Add2 : Sum
  Add3 : Sum  Inputs=+-
  Add4 : Sum  Inputs=+-
  Add5 : Sum  Inputs=+-
  Constant1 : Constant  Value=0  OutDataTypeStr=double
  Constant12 : Constant  Value=0  OutDataTypeStr=double
  Constant13 : Constant  Value=10  OutDataTypeStr=double
  Constant14 : Constant  Value=1000  OutDataTypeStr=double
  Constant17 : Constant  OutDataTypeStr=double
  Constant2 : Constant  Value=0.000001  OutDataTypeStr=double
  Divide{5..6,8,10} (4 alike) : Product  Inputs=**
  Divide7 : Product  Inputs=*/
  Divide9 : Product  Inputs=*/
  Gain : Gain  Gain=1/5000
  Gain1 : Gain  Gain=0.005
  Gain5 : Gain  Gain=0.005
  Mux2 : Mux  Inputs=2
  PI-ID3 : Subsystem  mask{ermax=0.5*pi, ermin=-0.5*pi, max=500, min=-500}
      mask prompts: ermax "Err max limit"; ermin "Err min limit"; max "Output max limit"; min "Output min limit"
  RC filter3 : Subsystem  mask{a=0.8}
      mask prompts: a "Time Constant"
  Scope1 : Scope
  Scope2 : Scope
  Sqrt : Sqrt  SaturateOnIntegerOverflow=on
  Switch1 : Switch  Criteria=u2 ~= 0
  Trigonometric Function : Trigonometry
  Trigonometric Function1 : Trigonometry  Operator=cos
  Unit Delay1 : UnitDelay  SampleTime=-1
  Unit Delay5 : UnitDelay  SampleTime=-1
  angle generation : Subsystem
  sin : Outport
  cos : Outport  Port=2
  angle_0 : Outport  Port=3
  tag scope: w1=global
  wires:
  belta/1 -> Add3/1
  Add3/1 -> Divide5/1, Divide5/2, Divide7/1
  Gain5/1 -> Add3/2
  Gain1/1 -> Add4/2
  Is_β/1 -> Gain5/1
  Is_α/1 -> Gain1/1
  Add4/1 -> Divide6/1, Divide6/2, Divide9/1
  Divide5/1 -> Add2/1
  Divide6/1 -> Add2/2
  Add2/1 -> Sqrt/1
  Divide7/1 -> sin/1, Divide8/2
  Divide9/1 -> cos/1, Divide10/1
  Trigonometric Function/1 -> Divide10/2
  Divide8/1 -> Add5/1, Mux2/1
  Divide10/1 -> Add5/2, Mux2/2
  Add5/1 -> PI-ID3/1(err), Scope2/1
  Constant17/1 -> PI-ID3/2(reset)
  Constant12/1 -> PI-ID3/5(D)
  Constant1/1 -> PI-ID3/6(OV)
  Constant14/1 -> PI-ID3/3(P)
  Constant13/1 -> PI-ID3/4(I)
  Gain/1 -> angle generation/1(freq)
  PI-ID3/1(out) -> Gain/1, RC filter3/1(x)
  angle generation/1(angle_0) -> angle_0/1, Unit Delay5/1, Unit Delay1/1
  Unit Delay5/1 -> Trigonometric Function1/1
  Unit Delay1/1 -> Trigonometric Function/1
  Trigonometric Function1/1 -> Divide8/1
  Sqrt/1 -> Switch1/2, Switch1/1
  Constant2/1 -> Switch1/3
  Switch1/1 -> Divide7/2, Divide9/2
  RC filter3/1(y) -> [w1]
  alpha/1 -> Add4/1
  Mux2/1 -> Scope1/1

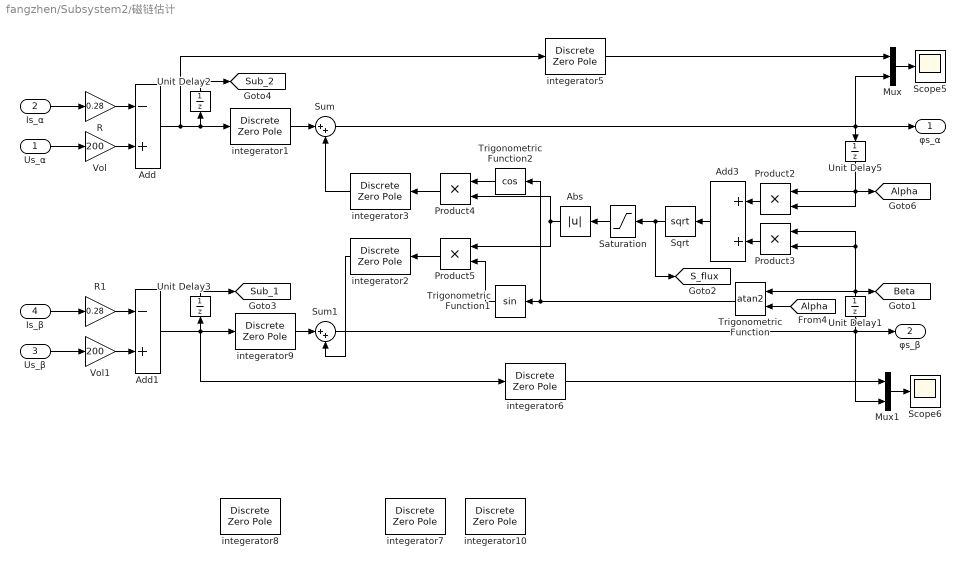
== system fangzhen/Subsystem2/磁链估计 ==
  Us_α : Inport
  Is_α : Inport  Port=2
  Us_β : Inport  Port=3
  Is_β : Inport  Port=4
  Abs : Abs
  Add : Sum  Inputs=-+
  Add1 : Sum  Inputs=-+
  Add3 : Sum
  Mux : Mux  Inputs=2
  Mux1 : Mux  Inputs=2
  Product{2..5} (4 alike) : Product  RndMeth=Zero
  R : Gain  Gain=0.28
  R1 : Gain  Gain=0.28
  Saturation : Saturate  UpperLimit=0.58  LowerLimit=-0.58
  Scope5 : Scope
  Scope6 : Scope
  Sqrt : Sqrt  SaturateOnIntegerOverflow=on
  Sum : Sum  Inputs=|++
  Sum1 : Sum  Inputs=|++
  Trigonometric Function : Trigonometry  Operator=atan2
  Trigonometric Function1 : Trigonometry
  Trigonometric Function2 : Trigonometry  Operator=cos
  Unit Delay{1..3,5} (4 alike) : UnitDelay  SampleTime=-1
  Vol : Gain  Gain=200
  Vol1 : Gain  Gain=200
  integerator1 : DiscreteZeroPole  Zeros=[0]  Poles=[1/1.03]  Gain=0.0002/1.03  SampleTime=-1
  integerator10 : DiscreteZeroPole  Zeros=[0]  Poles=[1/1.005]  Gain=0.0002/1.005*25  SampleTime=-1
  integerator2 : DiscreteZeroPole  Zeros=[0]  Poles=[1/1.03]  Gain=0.0002/1.03*150  SampleTime=-1
  integerator3 : DiscreteZeroPole  Zeros=[0]  Poles=[1/1.03]  Gain=0.0002/1.03*150  SampleTime=-1
  integerator5 : DiscreteZeroPole  Zeros=[0]  Poles=[1/1.0002]  Gain=0.0002/1.0002  SampleTime=-1
  integerator6 : DiscreteZeroPole  Zeros=[0]  Poles=[1/1.0002]  Gain=0.0002/1.0002  SampleTime=-1
  integerator7 : DiscreteZeroPole  Zeros=[0]  Poles=[1/1.05]  Gain=0.0002/1.05*250  SampleTime=-1
  integerator8 : DiscreteZeroPole  Zeros=[0]  Poles=[1/1.05]  Gain=0.0002/1.05  SampleTime=-1
  integerator9 : DiscreteZeroPole  Zeros=[0]  Poles=[1/1.03]  Gain=0.0002/1.03  SampleTime=-1
  φs_α : Outport
  φs_β : Outport  Port=2
  tag scope: Alpha=global, Beta=global, S_flux=global, Sub_1=global, Sub_2=global
  wires:
  Vol/1 -> Add/2
  Add/1 -> Unit Delay2/1, integerator1/1, integerator5/1
  Us_α/1 -> Vol/1
  Is_α/1 -> R/1
  R/1 -> Add/1
  R1/1 -> Add1/1
  Is_β/1 -> R1/1
  Us_β/1 -> Vol1/1
  Add1/1 -> Unit Delay3/1, integerator6/1, integerator9/1
  Vol1/1 -> Add1/2
  integerator1/1 -> Sum/1
  integerator9/1 -> Sum1/1
  Sum/1 -> Unit Delay5/1, Mux/2, φs_α/1
  Sum1/1 -> Unit Delay1/1, Mux1/2, φs_β/1
  Product3/1 -> Add3/2
  Product2/1 -> Add3/1
  Add3/1 -> Sqrt/1
  Product4/1 -> integerator3/1
  Product5/1 -> integerator2/1
  Abs/1 -> Product4/2, Product5/1
  Unit Delay1/1 -> [Beta], Product3/1, Product3/2, Trigonometric Function/1
  Unit Delay5/1 -> Product2/2, Product2/1, [Alpha]
  Unit Delay2/1 -> [Sub_2]
  Unit Delay3/1 -> [Sub_1]
  Sqrt/1 -> Saturation/1, [S_flux]
  Saturation/1 -> Abs/1
  [Alpha] -> Trigonometric Function/2
  Trigonometric Function/1 -> Trigonometric Function1/1, Trigonometric Function2/1
  Trigonometric Function1/1 -> Product5/2
  Trigonometric Function2/1 -> Product4/1
  integerator5/1 -> Mux/1
  Mux/1 -> Scope5/1
  Mux1/1 -> Scope6/1
  integerator2/1 -> Sum1/2
  integerator3/1 -> Sum/2
  integerator6/1 -> Mux1/1

== system fangzhen/Subsystem2/转速估计 ==
  Sub_1 : Inport
  Sub_2 : Inport  Port=2
  Alpha : Inport  Port=3
  Beta : Inport  Port=4
  Add : Sum  Inputs=+-
  Add1 : Sum
  Constant : Constant  Value=0.00001
  Divide{,1,3..4} (4 alike) : Product  Inputs=**
  Divide2 : Product  Inputs=*/
  Switch : Switch  Criteria=u2 > Threshold
  wr_c : Outport
  wires:
  Sub_1/1 -> Divide/1
  Alpha/1 -> Divide/2, Divide4/1, Divide4/2
  Sub_2/1 -> Divide1/1
  Beta/1 -> Divide1/2, Divide3/1, Divide3/2
  Divide/1 -> Add/1
  Divide1/1 -> Add/2
  Add/1 -> Divide2/1
  Divide3/1 -> Add1/1
  Divide4/1 -> Add1/2
  Divide2/1 -> wr_c/1
  Add1/1 -> Switch/2, Switch/1
  Switch/1 -> Divide2/2
  Constant/1 -> Switch/3

== system fangzhen/Subsystem2/PI-ID/RC filter8 ==
  x : Inport
  Constant2 : Constant  Value=a  OutDataTypeStr=double
  Constant3 : Constant  Value=1-a  OutDataTypeStr=double
  Divide : Product
  Divide1 : Product
  Sum2 : Sum
  Unit Delay2 : UnitDelay  SampleTime=-1
  y : Outport
  wires:
  Unit Delay2/1 -> Divide1/2
  Sum2/1 -> Unit Delay2/1, y/1
  Divide1/1 -> Sum2/2
  Divide/1 -> Sum2/1
  Constant3/1 -> Divide1/1
  Constant2/1 -> Divide/2
  x/1 -> Divide/1

== system fangzhen/Subsystem2/PI-ID2/RC filter8 ==
  x : Inport
  Constant2 : Constant  Value=a  OutDataTypeStr=double
  Constant3 : Constant  Value=1-a  OutDataTypeStr=double
  Divide : Product
  Divide1 : Product
  Sum2 : Sum
  Unit Delay2 : UnitDelay  SampleTime=-1
  y : Outport
  wires:
  x/1 -> Divide/1
  Constant2/1 -> Divide/2
  Constant3/1 -> Divide1/1
  Divide/1 -> Sum2/1
  Divide1/1 -> Sum2/2
  Sum2/1 -> y/1, Unit Delay2/1
  Unit Delay2/1 -> Divide1/2

== system fangzhen/Subsystem2/PI-IQ/RC filter8 ==
  x : Inport
  Constant2 : Constant  Value=a  OutDataTypeStr=double
  Constant3 : Constant  Value=1-a  OutDataTypeStr=double
  Divide : Product
  Divide1 : Product
  Sum2 : Sum
  Unit Delay2 : UnitDelay  SampleTime=-1
  y : Outport
  wires:
  x/1 -> Divide/1
  Constant2/1 -> Divide/2
  Constant3/1 -> Divide1/1
  Divide/1 -> Sum2/1
  Divide1/1 -> Sum2/2
  Sum2/1 -> y/1, Unit Delay2/1
  Unit Delay2/1 -> Divide1/2

== system fangzhen/Subsystem2/SPWM/Clarke1 ==
  In1 : Inport
  In2 : Inport  Port=2
  Constant58 : Constant  Value=3  OutDataTypeStr=double
  Divide : Product  Inputs=*/
  Gain : Gain  Gain=2
  Gain1 : Gain
  Gain2 : Gain
  Sqrt : Sqrt  SaturateOnIntegerOverflow=on
  Sum : Sum
  alpha : Outport
  beta : Outport  Port=2
  wires:
  Divide/1 -> Gain2/1
  Sqrt/1 -> Divide/2
  Constant58/1 -> Sqrt/1
  Sum/1 -> Divide/1
  Gain/1 -> Sum/2
  In1/1 -> Sum/1, Gain1/1
  In2/1 -> Gain/1
  Gain1/1 -> alpha/1
  Gain2/1 -> beta/1

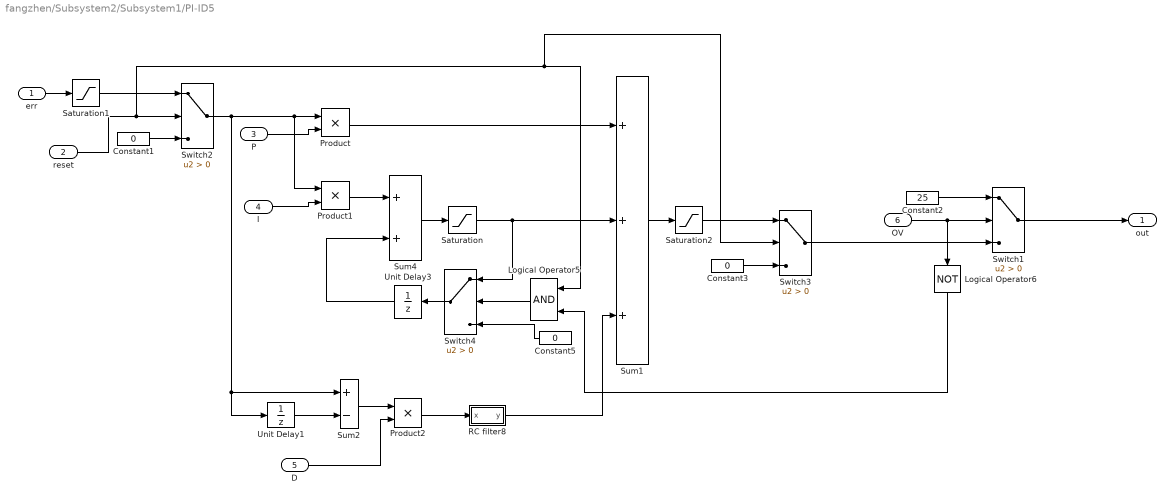
== system fangzhen/Subsystem2/Subsystem1/PI-ID5 ==
  err : Inport
  reset : Inport  Port=2
  P : Inport  Port=3
  I : Inport  Port=4
  D : Inport  Port=5
  OV : Inport  Port=6
  Constant1 : Constant  Value=0  OutDataTypeStr=Inherit: Inherit via back propagation
  Constant2 : Constant  Value=25  OutDataTypeStr=Inherit: Inherit via back propagation
  Constant3 : Constant  Value=0  OutDataTypeStr=Inherit: Inherit via back propagation
  Constant5 : Constant  Value=0  OutDataTypeStr=Inherit: Inherit via back propagation
  Logical Operator5 : Logic  AllPortsSameDT=off  OutDataTypeStr=boolean
  Logical Operator6 : Logic  Operator=NOT  AllPortsSameDT=off  OutDataTypeStr=boolean
  Product : Product  RndMeth=Zero
  Product1 : Product  RndMeth=Zero
  Product2 : Product  RndMeth=Zero
  RC filter8 : Subsystem  mask{a=0.4}
      mask prompts: a "Time Constant"
  Saturation : Saturate  UpperLimit=max  LowerLimit=min  LinearizeAsGain=off  ZeroCross=off  OutDataTypeStr=double
  Saturation1 : Saturate  UpperLimit=ermax  LowerLimit=ermin  LinearizeAsGain=off  ZeroCross=off  OutDataTypeStr=double
  Saturation2 : Saturate  UpperLimit=max  LowerLimit=min  LinearizeAsGain=off  ZeroCross=off  OutDataTypeStr=double
  Sum1 : Sum  Inputs=+++
  Sum2 : Sum  Inputs=+-
  Sum4 : Sum
  Switch{1..4} (4 alike) : Switch  Criteria=u2 > Threshold  SaturateOnIntegerOverflow=on  InputSameDT=on
  Unit Delay1 : UnitDelay  SampleTime=-1
  Unit Delay3 : UnitDelay  SampleTime=-1
  out : Outport
  wires:
  Logical Operator6/1 -> Logical Operator5/2
  Logical Operator5/1 -> Switch4/2
  RC filter8/1(y) -> Sum1/3
  Constant3/1 -> Switch3/3
  Switch3/1 -> Switch1/3
  Saturation2/1 -> Switch3/1
  Switch1/1 -> out/1
  OV/1 -> Logical Operator6/1, Switch1/2
  Constant2/1 -> Switch1/1
  Sum1/1 -> Saturation2/1
  Product2/1 -> RC filter8/1(x)
  Unit Delay1/1 -> Sum2/2
  D/1 -> Product2/2
  Sum2/1 -> Product2/1
  Switch4/1 -> Unit Delay3/1
  Unit Delay3/1 -> Sum4/2
  Saturation/1 -> Switch4/1, Sum1/2
  Sum4/1 -> Saturation/1
  Product1/1 -> Sum4/1
  I/1 -> Product1/2
  Product/1 -> Sum1/1
  Saturation1/1 -> Switch2/1
  err/1 -> Saturation1/1
  Constant1/1 -> Switch2/3
  reset/1 -> Logical Operator5/1, Switch3/2, Switch2/2
  Switch2/1 -> Unit Delay1/1, Sum2/1, Product1/1, Product/1
  P/1 -> Product/2
  Constant5/1 -> Switch4/3

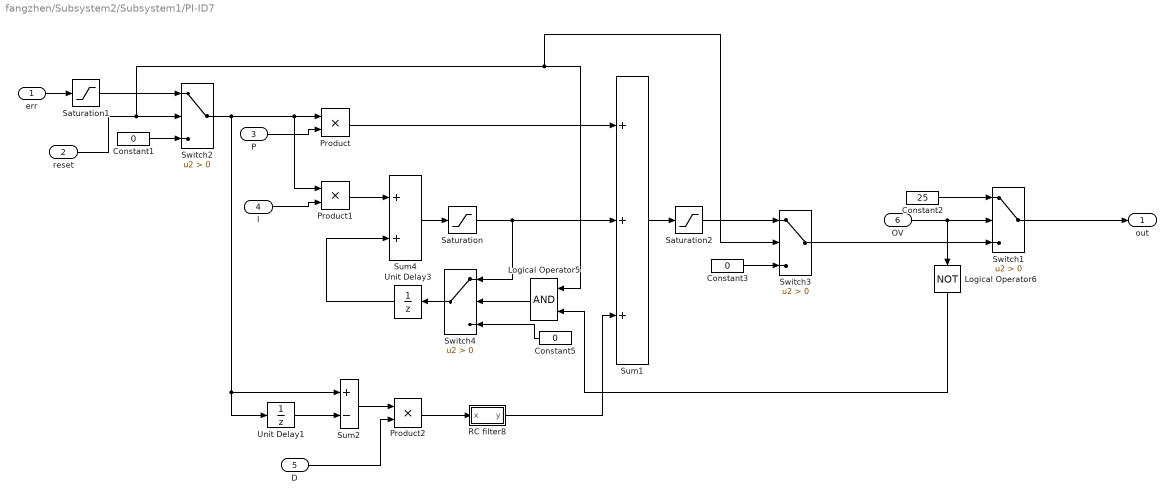
== system fangzhen/Subsystem2/Subsystem1/PI-ID7 ==
  err : Inport
  reset : Inport  Port=2
  P : Inport  Port=3
  I : Inport  Port=4
  D : Inport  Port=5
  OV : Inport  Port=6
  Constant1 : Constant  Value=0  OutDataTypeStr=Inherit: Inherit via back propagation
  Constant2 : Constant  Value=25  OutDataTypeStr=Inherit: Inherit via back propagation
  Constant3 : Constant  Value=0  OutDataTypeStr=Inherit: Inherit via back propagation
  Constant5 : Constant  Value=0  OutDataTypeStr=Inherit: Inherit via back propagation
  Logical Operator5 : Logic  AllPortsSameDT=off  OutDataTypeStr=boolean
  Logical Operator6 : Logic  Operator=NOT  AllPortsSameDT=off  OutDataTypeStr=boolean
  Product : Product  RndMeth=Zero
  Product1 : Product  RndMeth=Zero
  Product2 : Product  RndMeth=Zero
  RC filter8 : Subsystem  mask{a=0.4}
      mask prompts: a "Time Constant"
  Saturation : Saturate  UpperLimit=max  LowerLimit=min  LinearizeAsGain=off  ZeroCross=off  OutDataTypeStr=double
  Saturation1 : Saturate  UpperLimit=ermax  LowerLimit=ermin  LinearizeAsGain=off  ZeroCross=off  OutDataTypeStr=double
  Saturation2 : Saturate  UpperLimit=max  LowerLimit=min  LinearizeAsGain=off  ZeroCross=off  OutDataTypeStr=double
  Sum1 : Sum  Inputs=+++
  Sum2 : Sum  Inputs=+-
  Sum4 : Sum
  Switch{1..4} (4 alike) : Switch  Criteria=u2 > Threshold  SaturateOnIntegerOverflow=on  InputSameDT=on
  Unit Delay1 : UnitDelay  SampleTime=-1
  Unit Delay3 : UnitDelay  SampleTime=-1
  out : Outport
  wires:
  Logical Operator6/1 -> Logical Operator5/2
  Logical Operator5/1 -> Switch4/2
  RC filter8/1(y) -> Sum1/3
  Constant3/1 -> Switch3/3
  Switch3/1 -> Switch1/3
  Saturation2/1 -> Switch3/1
  Switch1/1 -> out/1
  OV/1 -> Logical Operator6/1, Switch1/2
  Constant2/1 -> Switch1/1
  Sum1/1 -> Saturation2/1
  Product2/1 -> RC filter8/1(x)
  Unit Delay1/1 -> Sum2/2
  D/1 -> Product2/2
  Sum2/1 -> Product2/1
  Switch4/1 -> Unit Delay3/1
  Unit Delay3/1 -> Sum4/2
  Saturation/1 -> Switch4/1, Sum1/2
  Sum4/1 -> Saturation/1
  Product1/1 -> Sum4/1
  I/1 -> Product1/2
  Product/1 -> Sum1/1
  Saturation1/1 -> Switch2/1
  err/1 -> Saturation1/1
  Constant1/1 -> Switch2/3
  reset/1 -> Logical Operator5/1, Switch3/2, Switch2/2
  Switch2/1 -> Unit Delay1/1, Sum2/1, Product1/1, Product/1
  P/1 -> Product/2
  Constant5/1 -> Switch4/3

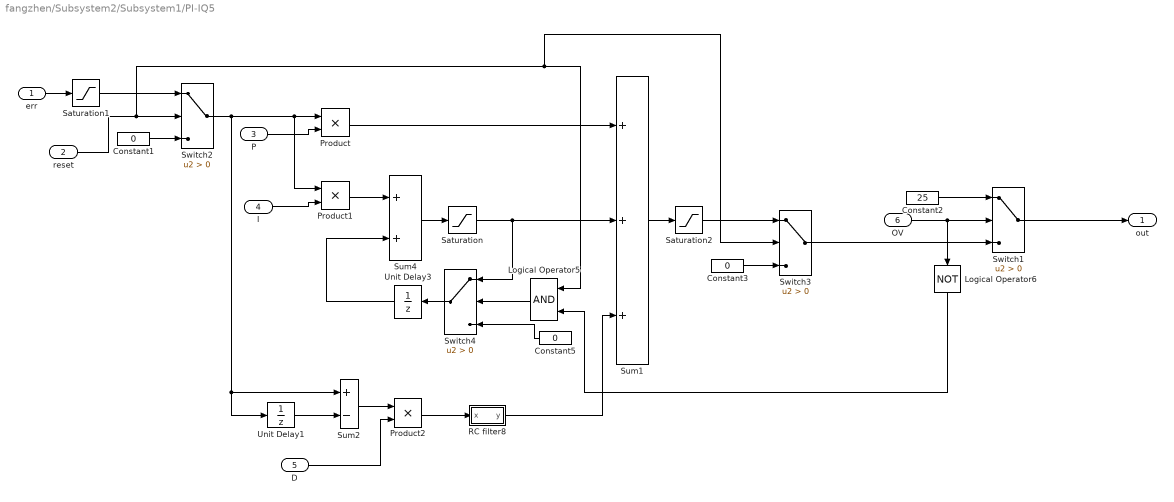
== system fangzhen/Subsystem2/Subsystem1/PI-IQ5 ==
  err : Inport
  reset : Inport  Port=2
  P : Inport  Port=3
  I : Inport  Port=4
  D : Inport  Port=5
  OV : Inport  Port=6
  Constant1 : Constant  Value=0  OutDataTypeStr=Inherit: Inherit via back propagation
  Constant2 : Constant  Value=25  OutDataTypeStr=Inherit: Inherit via back propagation
  Constant3 : Constant  Value=0  OutDataTypeStr=Inherit: Inherit via back propagation
  Constant5 : Constant  Value=0  OutDataTypeStr=Inherit: Inherit via back propagation
  Logical Operator5 : Logic  AllPortsSameDT=off  OutDataTypeStr=boolean
  Logical Operator6 : Logic  Operator=NOT  AllPortsSameDT=off  OutDataTypeStr=boolean
  Product : Product  RndMeth=Zero
  Product1 : Product  RndMeth=Zero
  Product2 : Product  RndMeth=Zero
  RC filter8 : Subsystem  mask{a=0.4}
      mask prompts: a "Time Constant"
  Saturation : Saturate  UpperLimit=max  LowerLimit=min  LinearizeAsGain=off  ZeroCross=off  OutDataTypeStr=double
  Saturation1 : Saturate  UpperLimit=ermax  LowerLimit=ermin  LinearizeAsGain=off  ZeroCross=off  OutDataTypeStr=double
  Saturation2 : Saturate  UpperLimit=max  LowerLimit=min  LinearizeAsGain=off  ZeroCross=off  OutDataTypeStr=double
  Sum1 : Sum  Inputs=+++
  Sum2 : Sum  Inputs=+-
  Sum4 : Sum
  Switch{1..4} (4 alike) : Switch  Criteria=u2 > Threshold  SaturateOnIntegerOverflow=on  InputSameDT=on
  Unit Delay1 : UnitDelay  SampleTime=-1
  Unit Delay3 : UnitDelay  SampleTime=-1
  out : Outport
  wires:
  Constant5/1 -> Switch4/3
  P/1 -> Product/2
  Switch2/1 -> Product/1, Product1/1, Sum2/1, Unit Delay1/1
  reset/1 -> Switch2/2, Switch3/2, Logical Operator5/1
  Constant1/1 -> Switch2/3
  err/1 -> Saturation1/1
  Saturation1/1 -> Switch2/1
  Product/1 -> Sum1/1
  I/1 -> Product1/2
  Product1/1 -> Sum4/1
  Sum4/1 -> Saturation/1
  Saturation/1 -> Sum1/2, Switch4/1
  Unit Delay3/1 -> Sum4/2
  Switch4/1 -> Unit Delay3/1
  Sum2/1 -> Product2/1
  D/1 -> Product2/2
  Unit Delay1/1 -> Sum2/2
  Product2/1 -> RC filter8/1(x)
  Sum1/1 -> Saturation2/1
  Constant2/1 -> Switch1/1
  OV/1 -> Switch1/2, Logical Operator6/1
  Switch1/1 -> out/1
  Saturation2/1 -> Switch3/1
  Switch3/1 -> Switch1/3
  Constant3/1 -> Switch3/3
  RC filter8/1(y) -> Sum1/3
  Logical Operator5/1 -> Switch4/2
  Logical Operator6/1 -> Logical Operator5/2

== system fangzhen/Subsystem2/Subsystem1/PI-IQ7 ==
  err : Inport
  reset : Inport  Port=2
  P : Inport  Port=3
  I : Inport  Port=4
  D : Inport  Port=5
  OV : Inport  Port=6
  Constant1 : Constant  Value=0  OutDataTypeStr=Inherit: Inherit via back propagation
  Constant2 : Constant  Value=25  OutDataTypeStr=Inherit: Inherit via back propagation
  Constant3 : Constant  Value=0  OutDataTypeStr=Inherit: Inherit via back propagation
  Constant5 : Constant  Value=0  OutDataTypeStr=Inherit: Inherit via back propagation
  Logical Operator5 : Logic  AllPortsSameDT=off  OutDataTypeStr=boolean
  Logical Operator6 : Logic  Operator=NOT  AllPortsSameDT=off  OutDataTypeStr=boolean
  Product : Product  RndMeth=Zero
  Product1 : Product  RndMeth=Zero
  Product2 : Product  RndMeth=Zero
  RC filter8 : Subsystem  mask{a=0.4}
      mask prompts: a "Time Constant"
  Saturation : Saturate  UpperLimit=max  LowerLimit=min  LinearizeAsGain=off  ZeroCross=off  OutDataTypeStr=double
  Saturation1 : Saturate  UpperLimit=ermax  LowerLimit=ermin  LinearizeAsGain=off  ZeroCross=off  OutDataTypeStr=double
  Saturation2 : Saturate  UpperLimit=max  LowerLimit=min  LinearizeAsGain=off  ZeroCross=off  OutDataTypeStr=double
  Sum1 : Sum  Inputs=+++
  Sum2 : Sum  Inputs=+-
  Sum4 : Sum
  Switch{1..4} (4 alike) : Switch  Criteria=u2 > Threshold  SaturateOnIntegerOverflow=on  InputSameDT=on
  Unit Delay1 : UnitDelay  SampleTime=-1
  Unit Delay3 : UnitDelay  SampleTime=-1
  out : Outport
  wires:
  Constant5/1 -> Switch4/3
  P/1 -> Product/2
  Switch2/1 -> Product/1, Product1/1, Sum2/1, Unit Delay1/1
  reset/1 -> Switch2/2, Switch3/2, Logical Operator5/1
  Constant1/1 -> Switch2/3
  err/1 -> Saturation1/1
  Saturation1/1 -> Switch2/1
  Product/1 -> Sum1/1
  I/1 -> Product1/2
  Product1/1 -> Sum4/1
  Sum4/1 -> Saturation/1
  Saturation/1 -> Sum1/2, Switch4/1
  Unit Delay3/1 -> Sum4/2
  Switch4/1 -> Unit Delay3/1
  Sum2/1 -> Product2/1
  D/1 -> Product2/2
  Unit Delay1/1 -> Sum2/2
  Product2/1 -> RC filter8/1(x)
  Sum1/1 -> Saturation2/1
  Constant2/1 -> Switch1/1
  OV/1 -> Switch1/2, Logical Operator6/1
  Switch1/1 -> out/1
  Saturation2/1 -> Switch3/1
  Switch3/1 -> Switch1/3
  Constant3/1 -> Switch3/3
  RC filter8/1(y) -> Sum1/3
  Logical Operator5/1 -> Switch4/2
  Logical Operator6/1 -> Logical Operator5/2

== system fangzhen/Subsystem2/Subsystem1/RC filter1 ==
  x : Inport
  Constant2 : Constant  Value=a  OutDataTypeStr=double
  Constant3 : Constant  Value=1-a  OutDataTypeStr=double
  Divide : Product
  Divide1 : Product
  Sum2 : Sum
  Unit Delay2 : UnitDelay  SampleTime=-1
  y : Outport
  wires:
  x/1 -> Divide/1
  Constant2/1 -> Divide/2
  Constant3/1 -> Divide1/1
  Divide/1 -> Sum2/1
  Divide1/1 -> Sum2/2
  Sum2/1 -> y/1, Unit Delay2/1
  Unit Delay2/1 -> Divide1/2

== system fangzhen/Subsystem2/Subsystem1/RC filter2 ==
  x : Inport
  Constant2 : Constant  Value=a  OutDataTypeStr=double
  Constant3 : Constant  Value=1-a  OutDataTypeStr=double
  Divide : Product
  Divide1 : Product
  Sum2 : Sum
  Unit Delay2 : UnitDelay  SampleTime=-1
  y : Outport
  wires:
  Unit Delay2/1 -> Divide1/2
  Sum2/1 -> Unit Delay2/1, y/1
  Divide1/1 -> Sum2/2
  Divide/1 -> Sum2/1
  Constant3/1 -> Divide1/1
  Constant2/1 -> Divide/2
  x/1 -> Divide/1

== system fangzhen/Subsystem2/Subsystem1/RC filter4 ==
  x : Inport
  Constant2 : Constant  Value=a  OutDataTypeStr=double
  Constant3 : Constant  Value=1-a  OutDataTypeStr=double
  Divide : Product
  Divide1 : Product
  Sum2 : Sum
  Unit Delay2 : UnitDelay  SampleTime=-1
  y : Outport
  wires:
  x/1 -> Divide/1
  Constant2/1 -> Divide/2
  Constant3/1 -> Divide1/1
  Divide/1 -> Sum2/1
  Divide1/1 -> Sum2/2
  Sum2/1 -> y/1, Unit Delay2/1
  Unit Delay2/1 -> Divide1/2

== system fangzhen/Subsystem2/Subsystem1/RC filter5 ==
  x : Inport
  Constant2 : Constant  Value=a  OutDataTypeStr=double
  Constant3 : Constant  Value=1-a  OutDataTypeStr=double
  Divide : Product
  Divide1 : Product
  Sum2 : Sum
  Unit Delay2 : UnitDelay  SampleTime=-1
  y : Outport
  wires:
  Unit Delay2/1 -> Divide1/2
  Sum2/1 -> Unit Delay2/1, y/1
  Divide1/1 -> Sum2/2
  Divide/1 -> Sum2/1
  Constant3/1 -> Divide1/1
  Constant2/1 -> Divide/2
  x/1 -> Divide/1
